simulink model "DriveLine"  (R2018a)
settings: Solver=VariableStepAuto  StartTime=0.0  StopTime=10.0  RelTol=1e-3
model workspace (MAT data in the model file):
  AccessoryLoad = 600
  C_ref = 600
  DrCycles.C505 = [0 1 2 3 4 5 6 7 8 9 10 11 ... (1012 elements, 506x2)]
  DrCycles.FTP = [0 1 2 3 4 5 6 7 8 9 10 11 ... (4956 elements, 2478x2)]
  DrCycles.UDDS = [0 1 2 3 4 5 6 7 8 9 10 11 ... (2746 elements, 1373x2)]
  DrCycles.HWFET = [0 1 2 3 4 5 6 7 8 9 10 11 ... (1532 elements, 766x2)]
  DrCycles.US06 = [0 1 2 3 4 5 6 7 8 9 10 11 ... (1194 elements, 597x2)]
  DrCycles.US06City = [0 1 2 3 4 5 6 7 8 9 10 11 ... (466 elements, 233x2)]
  DrCycles.US06Hwy = [0 1 2 3 4 5 6 7 8 9 10 11 ... (742 elements, 371x2)]
  K = 1.04716227018
  Kc_ref = 0.12
  Ki_ref = 0.01
  Kw_ref = 1.2e-05
  MDL.MotorModel.kc = 0.0452374100719
  MDL.MotorModel.ki = 0.0166666666667
  MDL.MotorModel.kw = 5.06640055941e-05
  MDL.MotorModel.C = 628.29736211
  MDL.MotorModel.MaxTrqOut = 500
  MDL.MotorModel.MaxPwrOut = 100000
  MDL.DrivelineModel.C0 = 600
  MDL.DrivelineModel.C1 = 0.012
  MDL.DrivelineModel.C2 = 4.9e-07
  MDL.DrivelineModel.G = 3.55
  MDL.DrivelineModel.Spinloss = 6
  MDL.DrivelineModel.Ftr_max = 5000
  MDL.DriverModel.Kp = 350
  MDL.DriverModel.Ki = 0
  MDL.DriverModel.Kd = 0
  MDL.DriverModel.BrakeGain = 100
  MDL.DriverModel.Ftr_Max = 5000
  MDL.DriverModel.Ptr_Max = 100000
  MDL.BrakeSys.MaxBrakeForce = 10000
  MDL.BrakeSys.RegenFraction = 0.55
  T_max = 500
  T_ref = 300
  TimeHWFET = 765
  TimeUDDS = 1372
  TimeUS06 = 596
  aeroDragCoeff = 0.38
  airDensity = 1.23
  energyCapacity = 12.6
  frontArea = 2.1
  gravity = 9.81
  inclinationAngle = 0
  inertialMassVeh = 2392
  initialSOC = 0.95
  internalResistance = 0.1
  massVeh = 2300
  openCircuitVoltage = 340
  rollingResistCoeff = 0.01
  w_max = 524
  w_ref = 834
  wheelRadius = 0.34
libraries: simulink x1
settings Model: Creator=100655384  LastModifiedBy=100655384

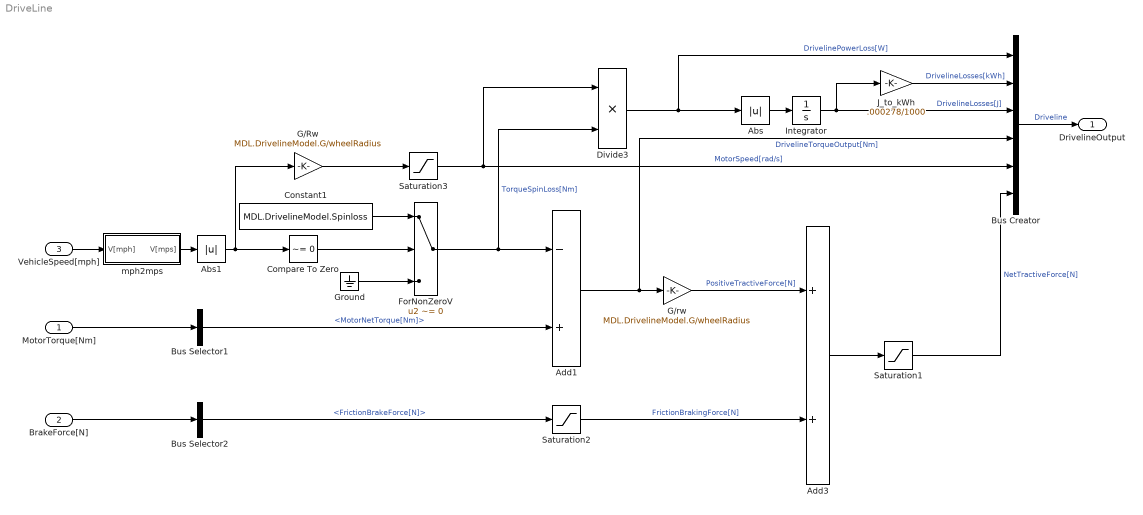
== system DriveLine ==
  MotorTorque[Nm] : Inport
  BrakeForce[N] : Inport  Port=2
  VehicleSpeed[mph] : Inport  Port=3
  Abs : Abs  ZeroCross=off
  Abs1 : Abs  ZeroCross=off
  Add1 : Sum  Inputs=-+
  Add3 : Sum
  Bus Creator : BusCreator  Inputs=6
  Bus Selector1 : BusSelector  OutputSignals=MotorNetTorque[Nm]
  Bus Selector2 : BusSelector  OutputSignals=FrictionBrakeForce[N]
  Compare To Zero : simulink/Logic and Bit Operations/Compare To Zero  relop=~=  OutDataTypeStr=boolean
  Constant1 : Constant  Value=MDL.DrivelineModel.Spinloss
  Divide3 : Product  Inputs=**
  ForNonZeroV : Switch  Criteria=u2 ~= 0  ZeroCross=off
  G/Rw : Gain  Gain=MDL.DrivelineModel.G/wheelRadius
  G/rw : Gain  Gain=MDL.DrivelineModel.G/wheelRadius
  Ground : Ground
  Integrator : Integrator  ZeroCross=off
  J_to_kWh : Gain  Gain=.000278/1000
  Saturation1 : Saturate  UpperLimit=5000  LowerLimit=-10000  ZeroCross=off
  Saturation2 : Saturate  UpperLimit=0  LowerLimit=-10000  ZeroCross=off
  Saturation3 : Saturate  UpperLimit=inf  LowerLimit=0.00001  ZeroCross=off
  mph2mps : Subsystem
  DrivelineOutput : Outport
  wires:
  Compare To Zero/1 -> ForNonZeroV/2
  Bus Selector1/1 -> Add1/2  "<MotorNetTorque[Nm]>"
  Integrator/1 -> J_to_kWh/1, Bus Creator/3  "DrivelineLosses[J]"
  J_to_kWh/1 -> Bus Creator/2  "DrivelineLosses[kWh]"
  Abs1/1 -> Compare To Zero/1, G/Rw/1
  Bus Creator/1 -> DrivelineOutput/1  "Driveline"
  Add3/1 -> Saturation1/1
  Bus Selector2/1 -> Saturation2/1  "<FrictionBrakeForce[N]>"
  Add1/1 -> Bus Creator/4, G/rw/1  "DrivelineTorqueOutput[Nm]"
  Constant1/1 -> ForNonZeroV/1
  mph2mps/1(V[mps]) -> Abs1/1
  MotorTorque[Nm]/1 -> Bus Selector1/1
  Saturation1/1 -> Bus Creator/6  "NetTractiveForce[N]"
  G/Rw/1 -> Saturation3/1
  Saturation3/1 -> Divide3/1, Bus Creator/5  "MotorSpeed[rad/s]"
  VehicleSpeed[mph]/1 -> mph2mps/1(V[mph])
  ForNonZeroV/1 -> Divide3/2, Add1/1  "TorqueSpinLoss[Nm]"
  BrakeForce[N]/1 -> Bus Selector2/1
  Saturation2/1 -> Add3/2  "FrictionBrakingForce[N]"
  Divide3/1 -> Bus Creator/1, Abs/1  "DrivelinePowerLoss[W]"
  Abs/1 -> Integrator/1
  G/rw/1 -> Add3/1  "PositiveTractiveForce[N]"
  Ground/1 -> ForNonZeroV/3

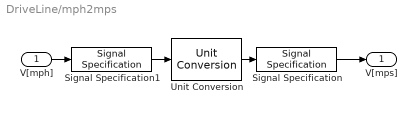
== system DriveLine/mph2mps ==
  V[mph] : Inport
  Signal Specification : SignalSpecification  Unit=m/s
  Signal Specification1 : SignalSpecification  Unit=mile/hr
  Unit Conversion : UnitConversion
  V[mps] : Outport
  wires:
  V[mph]/1 -> Signal Specification1/1
  Unit Conversion/1 -> Signal Specification/1
  Signal Specification1/1 -> Unit Conversion/1
  Signal Specification/1 -> V[mps]/1
